simulink model "ERLE"  (R2015a)
settings: Solver=ode45  StartTime=0.0  StopTime=1  RelTol=1e-3
libraries: dspstat3 x2
settings Model: Creator=Afonso  LastModifiedBy=Afonso

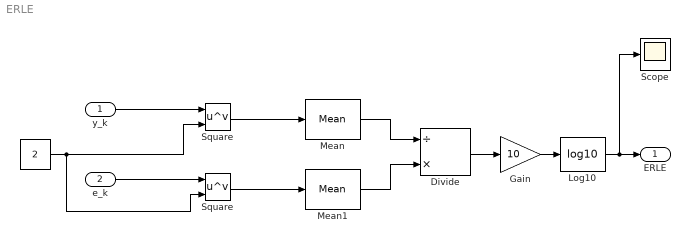
== system ERLE ==
  y_k : Inport
  e_k : Inport  Port=2
  " " : Constant  Value=2
  Divide : Product  Inputs=/*
  Gain : Gain  Gain=10
  Log10 : Math  Operator=log10  SaturateOnIntegerOverflow=on
  Mean : dspstat3/Mean  run=off  reset_popup=None  InputProcessing=Columns as channels (frame based)  directionMode=Each column  dimension=1  treatSBRowAsCol=on  roiEnable=off  roiType=Rectangles  roiPortion=Entire ROI  roiOutput=Individual statistics for each ROI  roiFlag=off  outputDataTypeStr=Inherit: Same as accumulator  outputLastDataTypeStr=Inherit: Same as accumulator  outputMin=[]  outputMax=[]  roundingMode=Floor  overflowMode=off
  Mean1 : dspstat3/Mean  run=off  reset_popup=None  InputProcessing=Columns as channels (frame based)  directionMode=Each column  dimension=1  treatSBRowAsCol=on  roiEnable=off  roiType=Rectangles  roiPortion=Entire ROI  roiOutput=Individual statistics for each ROI  roiFlag=off  outputDataTypeStr=Inherit: Same as accumulator  outputLastDataTypeStr=Inherit: Same as accumulator  outputMin=[]  outputMax=[]  roundingMode=Floor  overflowMode=off
  Scope : Scope
  Square : Math  Operator=pow  SaturateOnIntegerOverflow=on
  "Square " : Math  Operator=pow  SaturateOnIntegerOverflow=on
  ERLE : Outport
  wires:
  y_k/1 -> Square/1
  e_k/1 -> "Square "/1
  " "/1 -> "Square "/2, Square/2
  Square/1 -> Mean/1
  "Square "/1 -> Mean1/1
  Mean/1 -> Divide/1
  Mean1/1 -> Divide/2
  Divide/1 -> Gain/1
  Gain/1 -> Log10/1
  Log10/1 -> Scope/1, ERLE/1
